simulink model "DrawingWiiChuk"  (R2014a)
settings: Solver=ode3  StartTime=0.0  StopTime=inf  RelTol=1e-3
undefined symbols (not defined in the file): rpy2tr, serial
libraries: roblocks x6, instrumentlib x2, simulink x1
settings Model: Creator=Edoardo  LastModifiedBy=Edoardo
settings DebuggingCC: SolverPrmCheckMsg=none

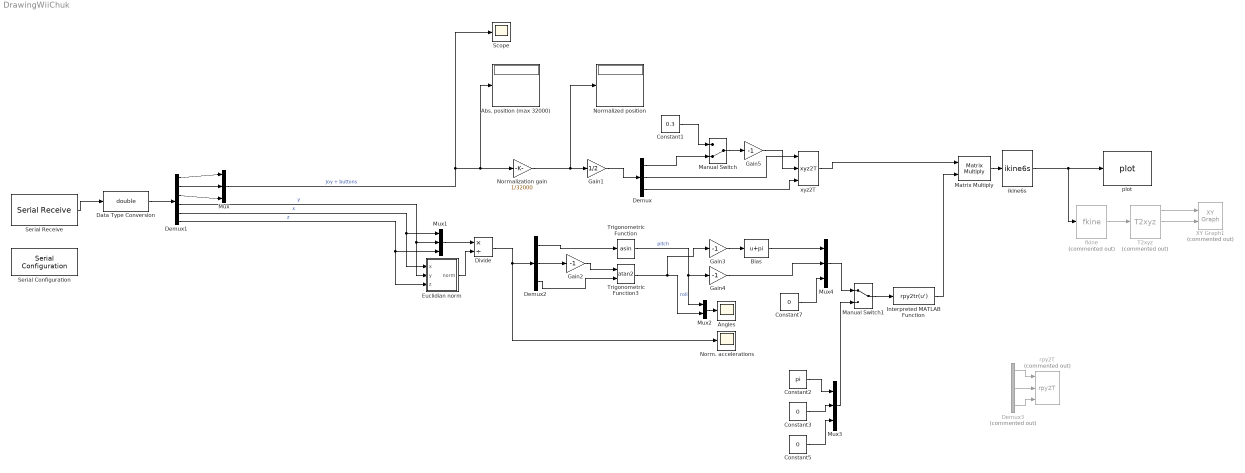
== system DrawingWiiChuk ==
  Abs. position (max 32000) : Display
  Angles : Scope
      settings: ShowLegends=on  YMin=-200  YMax=200  SaveName=ScopeData2
  Bias : Bias  Bias=pi
  Constant1 : Constant  Value=0.3
  Constant2 : Constant  Value=pi
  Constant3 : Constant  Value=0
  Constant5 : Constant  Value=0
  Constant7 : Constant  Value=0
  Data Type Conversion : DataTypeConversion  OutDataTypeStr=double
  Demux : Demux  Outputs=3
  Demux1 : Demux  Outputs=6
  Demux2 : Demux  Outputs=3
  Demux3 : Demux  Commented=on  Outputs=3
  Divide : Product  Inputs=*/
  Euclidian norm : Subsystem
  Gain1 : Gain  Gain=1/2
  Gain{2..5} (4 alike) : Gain  Gain=-1
  Interpreted MATLAB Function : MATLABFcn  MATLABFcn=rpy2tr(u')  OutputDimensions=[4 4]  OutputSignalType=real  Output1D=off
  Manual Switch : ManualSwitch  CurrentSetting=0
  Manual Switch1 : ManualSwitch
  Matrix Multiply : Product  Multiplication=Matrix(*)
  Mux{,1,3..4} (4 alike) : Mux  Inputs=3
  Mux2 : Mux  Inputs=2
  Norm. accelerations : Scope
      settings: ShowLegends=on  TimeRange=30  YMin=-1  YMax=1  SampleTime=0.01
  Normalization gain : Gain  Gain=1/32000
  Normalized position : Display
  Scope : Scope
      settings: YMin=-350  YMax=300
  Serial Configuration : instrumentlib/Serial Configuration  Priority=-200000  ComPortMenu=COM5  ComPort=COM5  ObjConstructor=serial('COM5');  BaudRate=115200  DataBits=8  Parity=none  StopBits=1  FlowControl=none  Timeout=10  ByteOrder=LittleEndian
  Serial Receive : instrumentlib/Serial Receive  ComPortMenu=COM5  ComPort=COM5  ObjConstructor=serial('COM5');  Terminator=<none>  DataSize="[6  1]"  DataType=int16  EnableBlockingMode=on  ActionDataUnavailable=Output last received value  CustomValue=120  SampleTime=0.01
  T2xyz : roblocks/Transform Conversion/T2xyz  Commented=on
  Trigonometric Function : Trigonometry  Operator=asin  OutputSignalType=real
  Trigonometric Function3 : Trigonometry  Operator=atan2  OutputSignalType=real
  XY Graph1 : simulink/Sinks/XY Graph  Commented=on  xmin=-1  xmax=1  ymin=-1  ymax=1  st=-1
  fkine : roblocks/Kinematics/fkine  Commented=on  robot=p560
  ikine6s : roblocks/Kinematics/ikine6s  robot=p560  conf='luf'
  plot : roblocks/Robot Graphics/plot  robot=p560  fps=25  holdplot=on
  rpy2T : roblocks/Transform Conversion/rpy2T  Commented=on
      link override MATLAB Fcn: MATLABFcn=rpy2tr(u')
  xyz2T : roblocks/Transform Conversion/xyz2T
  wires:
  ikine6s/1 -> plot/1, fkine/1
  fkine/1 -> T2xyz/1
  T2xyz/1 -> XY Graph1/1
  T2xyz/2 -> XY Graph1/2
  Demux/3 -> xyz2T/3
  Normalization gain/1 -> Normalized position/1, Gain1/1
  Gain1/1 -> Demux/1
  Demux/1 -> Manual Switch/2
  Constant1/1 -> Manual Switch/1
  Serial Receive/1 -> Data Type Conversion/1
  Mux/1 -> Scope/1, Abs. position (max 32000)/1, Normalization gain/1  "Joy + buttons"
  Demux1/1 -> Mux/1
  Demux1/2 -> Mux/2
  Demux1/3 -> Mux/3
  Demux1/5 -> Mux1/1, Euclidian norm/1(x)  "x"
  Demux1/6 -> Euclidian norm/3(z), Mux1/3  "z"
  Demux1/4 -> Mux1/2, Euclidian norm/2(y)  "y"
  Euclidian norm/1(norm) -> Divide/2
  Data Type Conversion/1 -> Demux1/1
  Mux1/1 -> Divide/1
  Divide/1 -> Demux2/1, Norm. accelerations/1
  Trigonometric Function/1 -> Gain4/1, Mux2/1  "pitch"
  Mux2/1 -> Angles/1
  Trigonometric Function3/1 -> Gain3/1, Mux2/2  "roll"
  Demux2/2 -> Gain2/1
  Gain2/1 -> Trigonometric Function3/1
  Demux2/3 -> Trigonometric Function3/2
  Demux2/1 -> Trigonometric Function/1
  Constant5/1 -> Mux3/3
  Matrix Multiply/1 -> ikine6s/1
  xyz2T/1 -> Matrix Multiply/1
  Constant3/1 -> Mux3/2
  Constant2/1 -> Mux3/1
  Demux3/2 -> rpy2T/2
  Demux3/1 -> rpy2T/1
  Demux3/3 -> rpy2T/3
  Interpreted MATLAB Function/1 -> Matrix Multiply/2
  Constant7/1 -> Mux4/3
  Manual Switch1/1 -> Interpreted MATLAB Function/1
  Mux3/1 -> Manual Switch1/2
  Mux4/1 -> Manual Switch1/1
  Bias/1 -> Mux4/1
  Gain3/1 -> Bias/1
  Gain4/1 -> Mux4/2
  Demux/2 -> xyz2T/1
  Manual Switch/1 -> Gain5/1
  Gain5/1 -> xyz2T/2

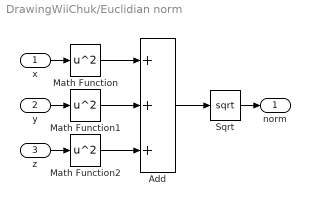
== system DrawingWiiChuk/Euclidian norm ==
  x : Inport
  y : Inport  Port=2
  z : Inport  Port=3
  Add : Sum  Inputs=+++
  Math Function : Math  Operator=square  SaturateOnIntegerOverflow=on
  Math Function1 : Math  Operator=square  SaturateOnIntegerOverflow=on
  Math Function2 : Math  Operator=square  SaturateOnIntegerOverflow=on
  Sqrt : Sqrt  SaturateOnIntegerOverflow=on
  norm : Outport
  wires:
  Math Function2/1 -> Add/3
  z/1 -> Math Function2/1
  Sqrt/1 -> norm/1
  Math Function1/1 -> Add/2
  Math Function/1 -> Add/1
  x/1 -> Math Function/1
  y/1 -> Math Function1/1
  Add/1 -> Sqrt/1
